simulink subsystem "RoboticArmGNC"  (R2023a)
settings: Solver=VariableStepAuto  StartTime=0.0  StopTime=10.0  RelTol=1e-3
undefined symbols (not defined in the file or in its folder): arm, ARM2_CONTROL_TYPE, jointControlData, nLink
libraries: simulink x1
settings Model: Creator=Andy  LastModifiedBy=Andy
settings OptimizationCC: ReuseModelBlockBuffer=off
settings ModelReferenceCC: EnableRefExpFcnMdlSchedulingChecks=on

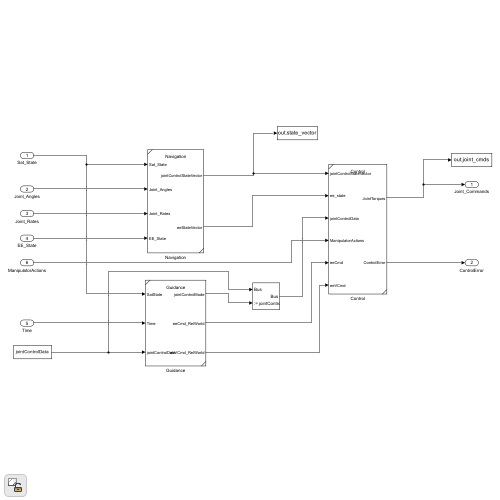
[thumbnail: Simulink's stored preview of the top-level diagram]
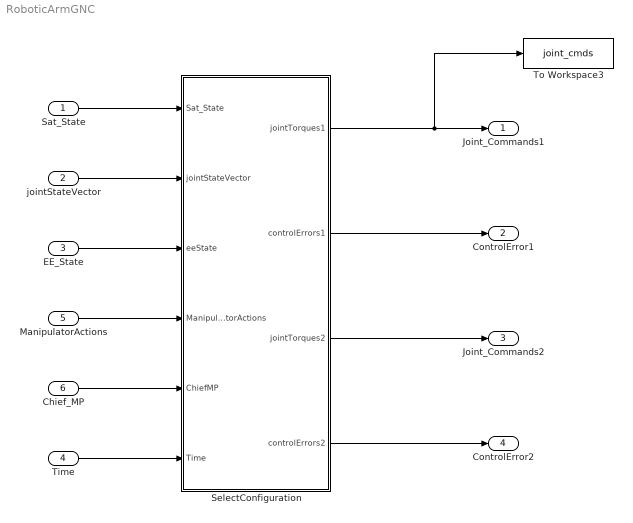
== system RoboticArmGNC ==
  Sat_State : Inport
  jointStateVector : Inport  Port=2
  EE_State : Inport  Port=3
  Time : Inport  Port=4
  ManipulatorActions : Inport  Port=5
  Chief_MP : Inport  Port=6
  SelectConfiguration : Subsystem  Variant=on
  To Workspace3 : ToWorkspace  VariableName=joint_cmds  SaveFormat=Timeseries  SampleTime=-1
  Joint_Commands1 : Outport
  ControlError1 : Outport  Port=2
  Joint_Commands2 : Outport  Port=3
  ControlError2 : Outport  Port=4
  wires:
  Sat_State/1 -> SelectConfiguration/1(Sat_State)
  Time/1 -> SelectConfiguration/6(Time)
  ManipulatorActions/1 -> SelectConfiguration/4(ManipulatorActions)
  SelectConfiguration/1(jointTorques1) -> Joint_Commands1/1, To Workspace3/1
  SelectConfiguration/3(jointTorques2) -> Joint_Commands2/1
  SelectConfiguration/4(controlErrors2) -> ControlError2/1
  SelectConfiguration/2(controlErrors1) -> ControlError1/1
  Chief_MP/1 -> SelectConfiguration/5(ChiefMP)
  jointStateVector/1 -> SelectConfiguration/2(jointStateVector)
  EE_State/1 -> SelectConfiguration/3(eeState)

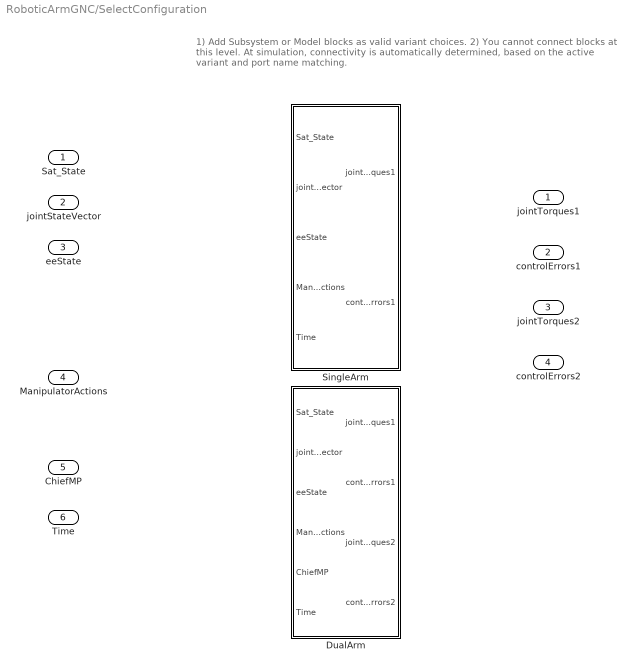
== system RoboticArmGNC/SelectConfiguration ==
  note: 1) Add Subsystem or Model blocks as valid variant choices.
      | 2) You cannot connect blocks at this level. At simulation, connectivity is automatically
      | determined, based on the active variant and port name matching.
  Sat_State : Inport
  jointStateVector : Inport  Port=2
  eeState : Inport  Port=3
  ManipulatorActions : Inport  Port=4
  ChiefMP : Inport  Port=5
  Time : Inport  Port=6
  DualArm : Subsystem  VariantControl=nARM==2
  SingleArm : Subsystem  VariantControl=nARM==1
  jointTorques1 : Outport
  controlErrors1 : Outport  Port=2
  jointTorques2 : Outport  Port=3
  controlErrors2 : Outport  Port=4

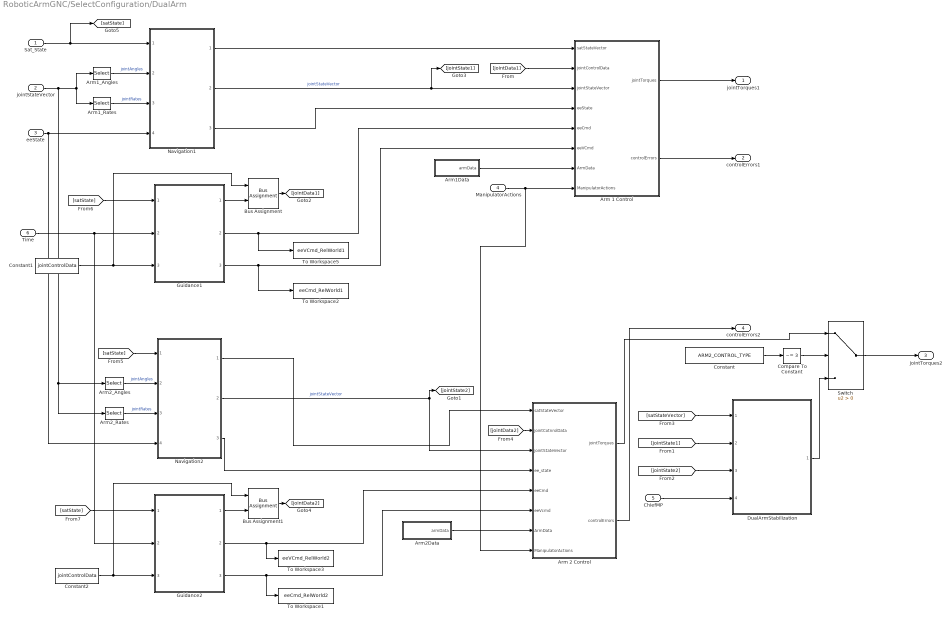
== system RoboticArmGNC/SelectConfiguration/DualArm ==
  Sat_State : Inport
  jointStateVector : Inport  Port=2
  eeState : Inport  Port=3
  ManipulatorActions : Inport  Port=4
  ChiefMP : Inport  Port=5
  Time : Inport  Port=6
  Arm 1 Control : Subsystem  Variant=on
  Arm 2 Control : Subsystem  Variant=on
  Arm1Data : Subsystem
  Arm1_Angles : Selector  IndexOptions=Index vector (dialog)  Indices=1:arm(1).nLink  OutputSizes=1
  Arm1_Rates : Selector  IndexOptions=Index vector (dialog)  Indices=1+arm(1).nLink+arm(2).nLink:2*arm(1).nLink+arm(2).nLink  OutputSizes=1
  Arm2Data : Subsystem
  Arm2_Angles : Selector  IndexOptions=Index vector (dialog)  Indices=1+arm(1).nLink:arm(1).nLink+arm(2).nLink  OutputSizes=1
  Arm2_Rates : Selector  IndexOptions=Index vector (dialog)  Indices=1+2*arm(1).nLink+arm(2).nLink:2*arm(1).nLink+2*arm(2).nLink  OutputSizes=1
  Bus Assignment : BusAssignment  AssignedSignals=jointControlMode
  Bus Assignment1 : BusAssignment  AssignedSignals=jointControlMode
  Compare To Constant : simulink/Logic and Bit Operations/Compare To Constant  relop=~=  const=3  OutDataTypeStr=boolean
  Constant : Constant  Value=ARM2_CONTROL_TYPE
  Constant1 : Constant  Value=jointControlData  OutDataTypeStr=Bus:jointControlDataBus
  Constant2 : Constant  Value=jointControlData  OutDataTypeStr=Bus:jointControlDataBus
  DualArmStabilization : Subsystem  VariantControl=VSS_DualArmStabilization  ReferencedSubsystem=DualArmStabilization
  Guidance1 : Subsystem  ReferencedSubsystem=Guidance
  Guidance2 : Subsystem  ReferencedSubsystem=Guidance
  Navigation1 : Subsystem  ReferencedSubsystem=Navigation
  Navigation2 : Subsystem  ReferencedSubsystem=Navigation
  Switch : Switch  Criteria=u2 > Threshold  SaturateOnIntegerOverflow=off  InputSameDT=off
  To Workspace1 : ToWorkspace  VariableName=eeCmd_RelWorld2  SaveFormat=Timeseries  SampleTime=-1
  To Workspace2 : ToWorkspace  VariableName=eeCmd_RelWorld1  SaveFormat=Timeseries  SampleTime=-1
  To Workspace3 : ToWorkspace  VariableName=eeVCmd_RelWorld2  SaveFormat=Timeseries  SampleTime=-1
  To Workspace5 : ToWorkspace  VariableName=eeVCmd_RelWorld1  SaveFormat=Timeseries  SampleTime=-1
  jointTorques1 : Outport
  controlErrors1 : Outport  Port=2
  jointTorques2 : Outport  Port=3
  controlErrors2 : Outport  Port=4
  wires:
  [satState] -> Guidance1/1
  [satState] -> Navigation2/1
  Guidance2/3 -> Arm 2 Control/6(eeVcmd), To Workspace1/1
  [jointData2] -> Arm 2 Control/2(jointCotnrolData)
  Bus Assignment1/1 -> [jointData2]
  Guidance2/1 -> Bus Assignment1/2
  Time/1 -> Guidance1/2, Guidance2/2
  Constant2/1 -> Guidance2/3, Bus Assignment1/1
  Guidance2/2 -> Arm 2 Control/5(eeCmd), To Workspace3/1
  [satState] -> Guidance2/1
  Constant1/1 -> Guidance1/3, Bus Assignment/1
  Sat_State/1 -> Navigation1/1, [satState]
  Guidance1/1 -> Bus Assignment/2
  Bus Assignment/1 -> [jointData1]
  Navigation2/3 -> Arm 2 Control/4(ee_state)
  eeState/1 -> Navigation1/4, Navigation2/4
  Navigation1/3 -> Arm 1 Control/4(eeState)
  Navigation1/1 -> Arm 1 Control/1(satStateVector)
  Navigation2/2 -> Arm 2 Control/3(jointStateVector), [jointState2]  "jointStateVector"
  Arm2_Rates/1 -> Navigation2/3  "jointRates"
  Arm2_Angles/1 -> Navigation2/2  "jointAngles"
  Arm1_Rates/1 -> Navigation1/3  "jointRates"
  Arm1_Angles/1 -> Navigation1/2  "jointAngles"
  [jointState2] -> DualArmStabilization/3
  [jointState1] -> DualArmStabilization/2
  ChiefMP/1 -> DualArmStabilization/4
  [satStateVector] -> DualArmStabilization/1
  Navigation2/1 -> Arm 2 Control/1(satStateVector)
  Compare To Constant/1 -> Switch/2
  Constant/1 -> Compare To Constant/1
  DualArmStabilization/1 -> Switch/3
  Arm 2 Control/1(jointTorques) -> Switch/1
  Switch/1 -> jointTorques2/1
  Arm 1 Control/1(jointTorques) -> jointTorques1/1
  Arm 2 Control/2(controlErrors) -> controlErrors2/1
  Arm 1 Control/2(controlErrors) -> controlErrors1/1
  [jointData1] -> Arm 1 Control/2(jointControlData)
  Arm1Data/1(armData) -> Arm 1 Control/7(ArmData)
  ManipulatorActions/1 -> Arm 1 Control/8(ManipulatorActions), Arm 2 Control/8(ManipulatorActions)
  Arm2Data/1(armData) -> Arm 2 Control/7(ArmData)
  Navigation1/2 -> [jointState1], Arm 1 Control/3(jointStateVector)  "jointStateVector"
  Guidance1/2 -> Arm 1 Control/5(eeCmd), To Workspace5/1
  jointStateVector/1 -> Arm2_Angles/1, Arm2_Rates/1, Arm1_Rates/1, Arm1_Angles/1
  Guidance1/3 -> Arm 1 Control/6(eeVCmd), To Workspace2/1

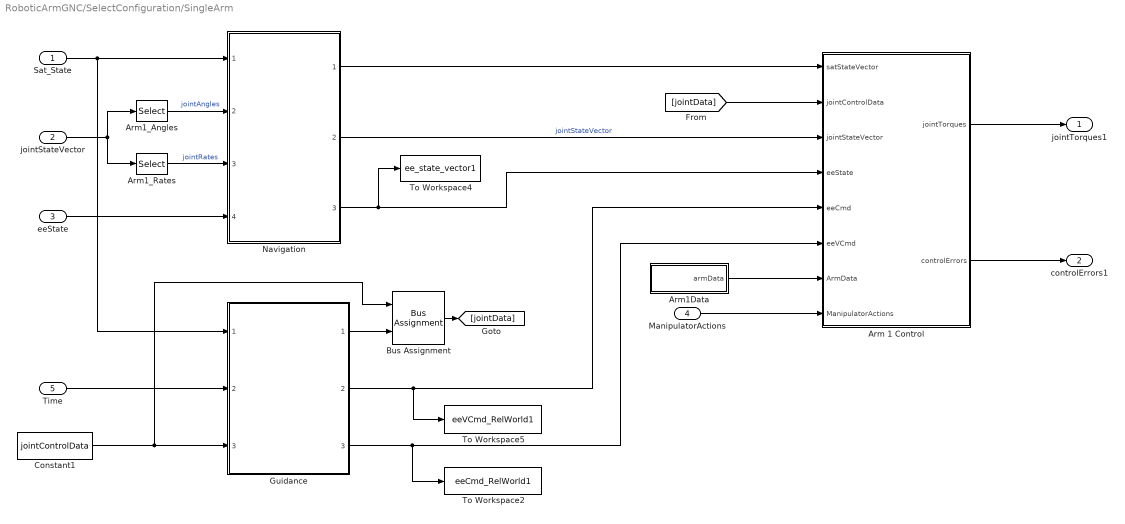
== system RoboticArmGNC/SelectConfiguration/SingleArm ==
  Sat_State : Inport
  jointStateVector : Inport  Port=2
  eeState : Inport  Port=3
  ManipulatorActions : Inport  Port=4
  Time : Inport  Port=5
  Arm 1 Control : Subsystem  Variant=on
  Arm1Data : Subsystem
  Arm1_Angles : Selector  IndexOptions=Index vector (dialog)  Indices=1:arm(1).nLink  OutputSizes=1
  Arm1_Rates : Selector  IndexOptions=Index vector (dialog)  Indices=1+arm(1).nLink+arm(2).nLink:2*arm(1).nLink+arm(2).nLink  OutputSizes=1
  Bus Assignment : BusAssignment  AssignedSignals=jointControlMode
  Constant1 : Constant  Value=jointControlData  OutDataTypeStr=Bus:jointControlDataBus
  Guidance : Subsystem  ReferencedSubsystem=Guidance
  Navigation : Subsystem  ReferencedSubsystem=Navigation
  To Workspace2 : ToWorkspace  VariableName=eeCmd_RelWorld1  SaveFormat=Timeseries  SampleTime=-1
  To Workspace4 : ToWorkspace  VariableName=ee_state_vector1  SaveFormat=Timeseries  SampleTime=-1
  To Workspace5 : ToWorkspace  VariableName=eeVCmd_RelWorld1  SaveFormat=Timeseries  SampleTime=-1
  jointTorques1 : Outport
  controlErrors1 : Outport  Port=2
  wires:
  [jointData] -> Arm 1 Control/2(jointControlData)
  Guidance/1 -> Bus Assignment/2
  Constant1/1 -> Guidance/3, Bus Assignment/1
  Time/1 -> Guidance/2
  Navigation/3 -> Arm 1 Control/4(eeState), To Workspace4/1
  eeState/1 -> Navigation/4
  Navigation/1 -> Arm 1 Control/1(satStateVector)
  Sat_State/1 -> Navigation/1, Guidance/1
  Arm1_Rates/1 -> Navigation/3  "jointRates"
  Arm1_Angles/1 -> Navigation/2  "jointAngles"
  Arm 1 Control/1(jointTorques) -> jointTorques1/1
  Arm 1 Control/2(controlErrors) -> controlErrors1/1
  Bus Assignment/1 -> [jointData]
  Arm1Data/1(armData) -> Arm 1 Control/7(ArmData)
  ManipulatorActions/1 -> Arm 1 Control/8(ManipulatorActions)
  Navigation/2 -> Arm 1 Control/3(jointStateVector)  "jointStateVector"
  Guidance/2 -> Arm 1 Control/5(eeCmd), To Workspace5/1
  jointStateVector/1 -> Arm1_Rates/1, Arm1_Angles/1
  Guidance/3 -> Arm 1 Control/6(eeVCmd), To Workspace2/1

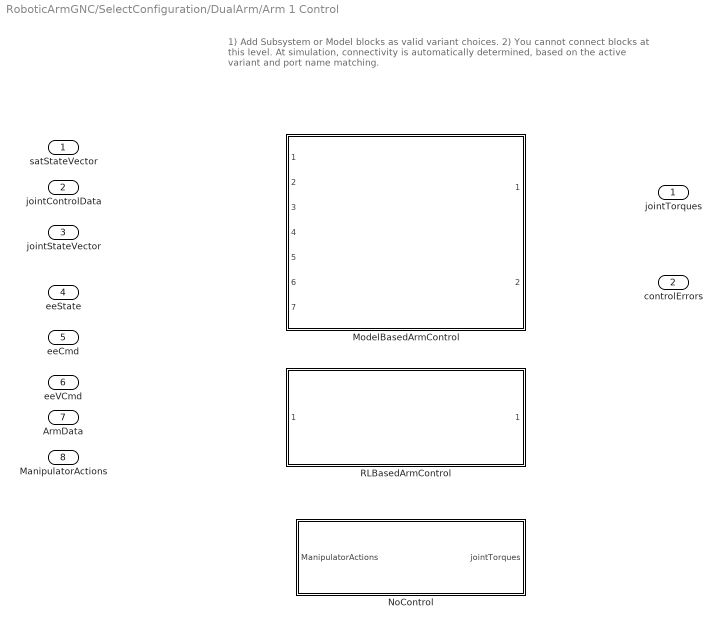
== system RoboticArmGNC/SelectConfiguration/DualArm/Arm 1 Control ==
  note: 1) Add Subsystem or Model blocks as valid variant choices.
      | 2) You cannot connect blocks at this level. At simulation, connectivity is automatically
      | determined, based on the active variant and port name matching.
  satStateVector : Inport
  jointControlData : Inport  Port=2
  jointStateVector : Inport  Port=3
  eeState : Inport  Port=4
  eeCmd : Inport  Port=5
  eeVCmd : Inport  Port=6
  ArmData : Inport  Port=7
  ManipulatorActions : Inport  Port=8
  ModelBasedArmControl : Subsystem  VariantControl=ARM1_CONTROL_TYPE == 1  ReferencedSubsystem=ModelBasedArmControl
  NoControl : Subsystem  VariantControl=(default)
  RLBasedArmControl : Subsystem  VariantControl=ARM1_CONTROL_TYPE == 2  ReferencedSubsystem=RLBasedArmControl
  jointTorques : Outport
  controlErrors : Outport  Port=2

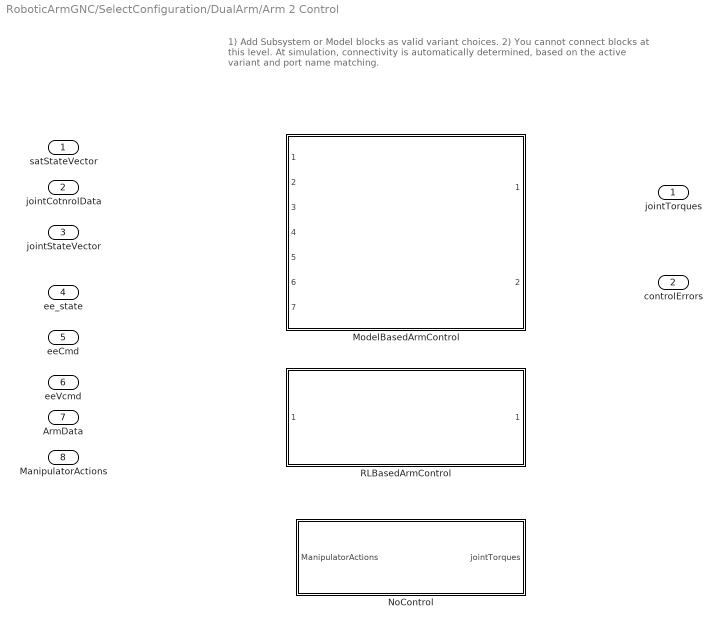
== system RoboticArmGNC/SelectConfiguration/DualArm/Arm 2 Control ==
  note: 1) Add Subsystem or Model blocks as valid variant choices.
      | 2) You cannot connect blocks at this level. At simulation, connectivity is automatically
      | determined, based on the active variant and port name matching.
  satStateVector : Inport
  jointCotnrolData : Inport  Port=2
  jointStateVector : Inport  Port=3
  ee_state : Inport  Port=4
  eeCmd : Inport  Port=5
  eeVcmd : Inport  Port=6
  ArmData : Inport  Port=7
  ManipulatorActions : Inport  Port=8
  ModelBasedArmControl : Subsystem  VariantControl=ARM2_CONTROL_TYPE == 1  ReferencedSubsystem=ModelBasedArmControl
  NoControl : Subsystem  VariantControl=(default)
  RLBasedArmControl : Subsystem  VariantControl=ARM2_CONTROL_TYPE == 2  ReferencedSubsystem=RLBasedArmControl
  jointTorques : Outport
  controlErrors : Outport  Port=2

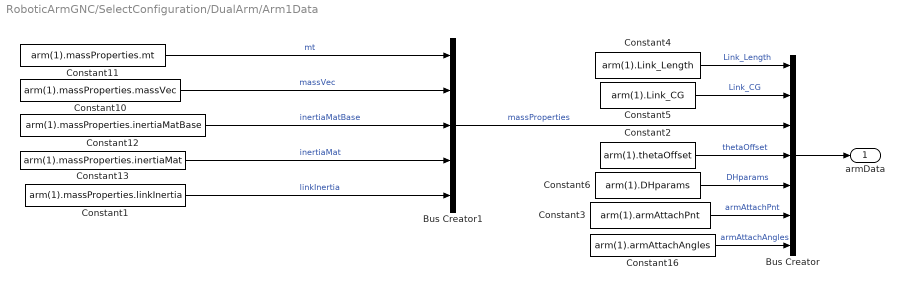
== system RoboticArmGNC/SelectConfiguration/DualArm/Arm1Data ==
  Bus Creator : BusCreator  Inputs=7
  Bus Creator1 : BusCreator  Inputs=5  OutDataTypeStr=Bus: MassPropertiesBus
      settings: InheritFromInputs=off
  Constant1 : Constant  Value=arm(1).massProperties.linkInertia
  Constant10 : Constant  Value=arm(1).massProperties.massVec
  Constant11 : Constant  Value=arm(1).massProperties.mt
  Constant12 : Constant  Value=arm(1).massProperties.inertiaMatBase
  Constant13 : Constant  Value=arm(1).massProperties.inertiaMat
  Constant16 : Constant  Value=arm(1).armAttachAngles
  Constant2 : Constant  Value=arm(1).thetaOffset
  Constant3 : Constant  Value=arm(1).armAttachPnt
  Constant4 : Constant  Value=arm(1).Link_Length
  Constant5 : Constant  Value=arm(1).Link_CG
  Constant6 : Constant  Value=arm(1).DHparams
  armData : Outport
  wires:
  Constant1/1 -> Bus Creator1/5  "linkInertia"
  Bus Creator/1 -> armData/1
  Constant16/1 -> Bus Creator/7  "armAttachAngles"
  Constant3/1 -> Bus Creator/6  "armAttachPnt"
  Constant4/1 -> Bus Creator/1  "Link_Length"
  Constant5/1 -> Bus Creator/2  "Link_CG"
  Constant6/1 -> Bus Creator/5  "DHparams"
  Constant2/1 -> Bus Creator/4  "thetaOffset"
  Constant12/1 -> Bus Creator1/3  "inertiaMatBase"
  Constant13/1 -> Bus Creator1/4  "inertiaMat"
  Constant10/1 -> Bus Creator1/2  "massVec"
  Constant11/1 -> Bus Creator1/1  "mt"
  Bus Creator1/1 -> Bus Creator/3  "massProperties"

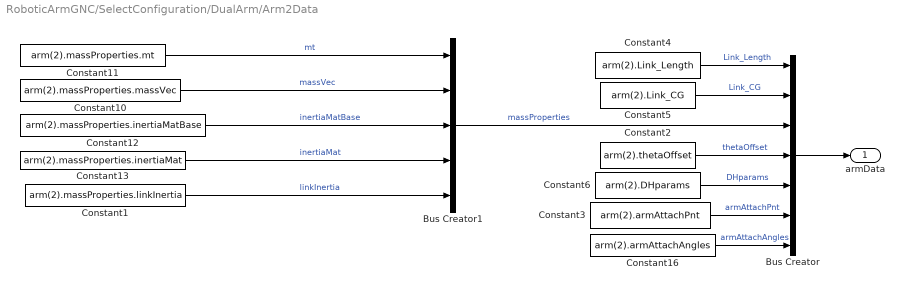
== system RoboticArmGNC/SelectConfiguration/DualArm/Arm2Data ==
  Bus Creator : BusCreator  Inputs=7
  Bus Creator1 : BusCreator  Inputs=5  OutDataTypeStr=Bus: MassPropertiesBus
      settings: InheritFromInputs=off
  Constant1 : Constant  Value=arm(2).massProperties.linkInertia
  Constant10 : Constant  Value=arm(2).massProperties.massVec
  Constant11 : Constant  Value=arm(2).massProperties.mt
  Constant12 : Constant  Value=arm(2).massProperties.inertiaMatBase
  Constant13 : Constant  Value=arm(2).massProperties.inertiaMat
  Constant16 : Constant  Value=arm(2).armAttachAngles
  Constant2 : Constant  Value=arm(2).thetaOffset
  Constant3 : Constant  Value=arm(2).armAttachPnt
  Constant4 : Constant  Value=arm(2).Link_Length
  Constant5 : Constant  Value=arm(2).Link_CG
  Constant6 : Constant  Value=arm(2).DHparams
  armData : Outport
  wires:
  Constant1/1 -> Bus Creator1/5  "linkInertia"
  Bus Creator/1 -> armData/1
  Constant16/1 -> Bus Creator/7  "armAttachAngles"
  Constant3/1 -> Bus Creator/6  "armAttachPnt"
  Constant4/1 -> Bus Creator/1  "Link_Length"
  Constant5/1 -> Bus Creator/2  "Link_CG"
  Constant6/1 -> Bus Creator/5  "DHparams"
  Constant2/1 -> Bus Creator/4  "thetaOffset"
  Constant12/1 -> Bus Creator1/3  "inertiaMatBase"
  Constant13/1 -> Bus Creator1/4  "inertiaMat"
  Constant10/1 -> Bus Creator1/2  "massVec"
  Constant11/1 -> Bus Creator1/1  "mt"
  Bus Creator1/1 -> Bus Creator/3  "massProperties"

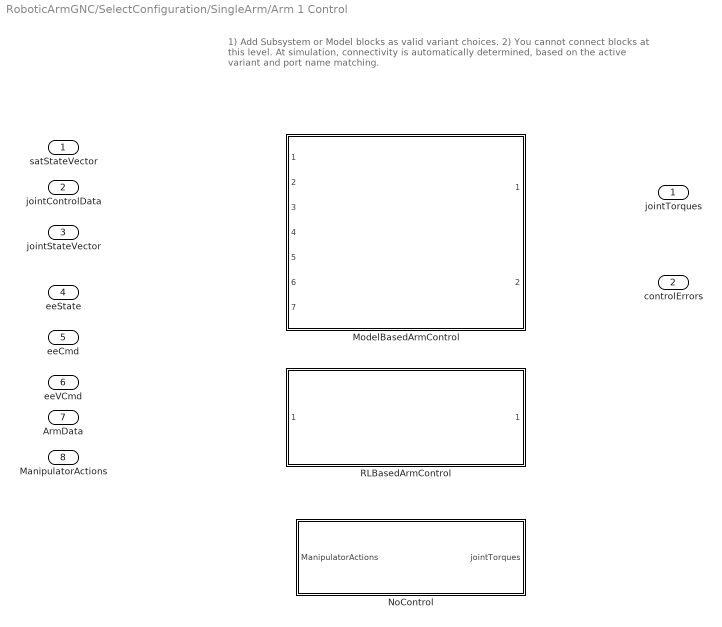
== system RoboticArmGNC/SelectConfiguration/SingleArm/Arm 1 Control ==
  note: 1) Add Subsystem or Model blocks as valid variant choices.
      | 2) You cannot connect blocks at this level. At simulation, connectivity is automatically
      | determined, based on the active variant and port name matching.
  satStateVector : Inport
  jointControlData : Inport  Port=2
  jointStateVector : Inport  Port=3
  eeState : Inport  Port=4
  eeCmd : Inport  Port=5
  eeVCmd : Inport  Port=6
  ArmData : Inport  Port=7
  ManipulatorActions : Inport  Port=8
  ModelBasedArmControl : Subsystem  VariantControl=ARM1_CONTROL_TYPE == 1  ReferencedSubsystem=ModelBasedArmControl
  NoControl : Subsystem  VariantControl=(default)
  RLBasedArmControl : Subsystem  VariantControl=ARM1_CONTROL_TYPE == 2  ReferencedSubsystem=RLBasedArmControl
  jointTorques : Outport
  controlErrors : Outport  Port=2

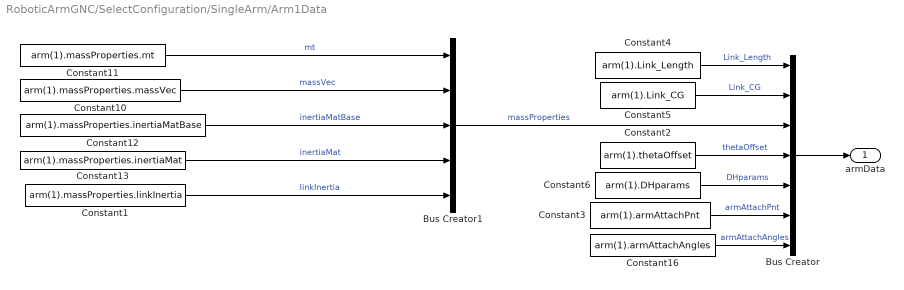
== system RoboticArmGNC/SelectConfiguration/SingleArm/Arm1Data ==
  Bus Creator : BusCreator  Inputs=7
  Bus Creator1 : BusCreator  Inputs=5  OutDataTypeStr=Bus: MassPropertiesBus
      settings: InheritFromInputs=off
  Constant1 : Constant  Value=arm(1).massProperties.linkInertia
  Constant10 : Constant  Value=arm(1).massProperties.massVec
  Constant11 : Constant  Value=arm(1).massProperties.mt
  Constant12 : Constant  Value=arm(1).massProperties.inertiaMatBase
  Constant13 : Constant  Value=arm(1).massProperties.inertiaMat
  Constant16 : Constant  Value=arm(1).armAttachAngles
  Constant2 : Constant  Value=arm(1).thetaOffset
  Constant3 : Constant  Value=arm(1).armAttachPnt
  Constant4 : Constant  Value=arm(1).Link_Length
  Constant5 : Constant  Value=arm(1).Link_CG
  Constant6 : Constant  Value=arm(1).DHparams
  armData : Outport
  wires:
  Constant1/1 -> Bus Creator1/5  "linkInertia"
  Bus Creator/1 -> armData/1
  Constant16/1 -> Bus Creator/7  "armAttachAngles"
  Constant3/1 -> Bus Creator/6  "armAttachPnt"
  Constant4/1 -> Bus Creator/1  "Link_Length"
  Constant5/1 -> Bus Creator/2  "Link_CG"
  Constant6/1 -> Bus Creator/5  "DHparams"
  Constant2/1 -> Bus Creator/4  "thetaOffset"
  Constant12/1 -> Bus Creator1/3  "inertiaMatBase"
  Constant13/1 -> Bus Creator1/4  "inertiaMat"
  Constant10/1 -> Bus Creator1/2  "massVec"
  Constant11/1 -> Bus Creator1/1  "mt"
  Bus Creator1/1 -> Bus Creator/3  "massProperties"

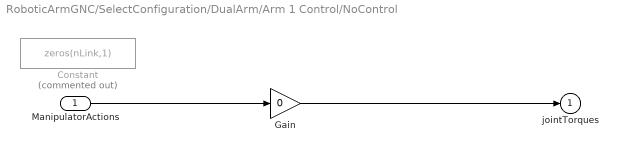
== system RoboticArmGNC/SelectConfiguration/DualArm/Arm 1 Control/NoControl ==
  ManipulatorActions : Inport
  Constant : Constant  Commented=on  Value=zeros(nLink,1)
  Gain : Gain  Gain=0
  jointTorques : Outport
  wires:
  Gain/1 -> jointTorques/1
  ManipulatorActions/1 -> Gain/1

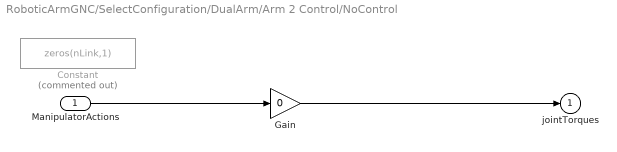
== system RoboticArmGNC/SelectConfiguration/DualArm/Arm 2 Control/NoControl ==
  ManipulatorActions : Inport
  Constant : Constant  Commented=on  Value=zeros(nLink,1)
  Gain : Gain  Gain=0
  jointTorques : Outport
  wires:
  ManipulatorActions/1 -> Gain/1
  Gain/1 -> jointTorques/1

== system RoboticArmGNC/SelectConfiguration/SingleArm/Arm 1 Control/NoControl ==
  ManipulatorActions : Inport
  Constant : Constant  Commented=on  Value=zeros(nLink,1)
  Gain : Gain  Gain=0
  jointTorques : Outport
  wires:
  Gain/1 -> jointTorques/1
  ManipulatorActions/1 -> Gain/1
